simulink model "versuch2_7_3"  (R2021a)
settings: Solver=ode3  StartTime=0.0  StopTime=50  FixedStep=0.01  RelTol=1e-3
StopFcn:
  | clear con
model workspace (MAT data in the model file):
  A = Simulink.Signal
  A.DataType = 'auto'
  A.Dimensions = 1
  A.DimensionsMode = 'auto'
  A.Complexity = 'auto'
  A.SampleTime = -1
  A.SamplingMode = 'auto'
undefined symbols (not defined in the file): sigbuilder_block
libraries: simulink x11, simulink_extras x6, aerolibanimutils x1, hdlsllib x1
(part 1 of 2)
settings Model: Creator=Jan  LastModifiedBy=Oceaner
settings SolverCC: AlgebraicLoopSolver=TrustRegion
settings DataIOCC: ReturnWorkspaceOutputs=off
settings DebuggingCC: SFMachineParentedDataDiag=warning  ArithmeticOperatorsInVariantConditions=warning
settings SFSimCC: SimUseLocalCustomCode=off  CustomCodeUndefinedFunction=UseInterfaceOnly
settings RTWCC: RTWUseLocalCustomCode=off
settings CodeAppCC: StateflowObjectComments=on
settings SimscapeCC: SimscapeNormalizeSystem=off

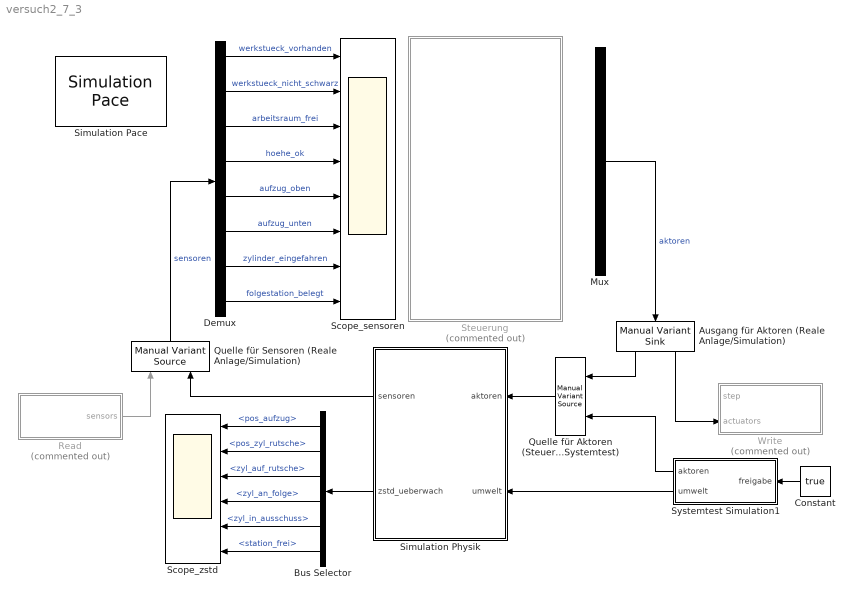
== system versuch2_7_3 ==
  " Scope_zstd" : Scope  NumInputPorts=6
  Ausgang für Aktoren (Reale Anlage/Simulation) : simulink/Signal Routing/Manual Variant Sink  NumChoices=2  LabelModeActiveChoice=V_1
  Bus Selector : BusSelector  OutputSignals=pos_aufzug,pos_zyl_rutsche,zyl_auf_rutsche,zyl_an_folge,zyl_in_ausschuss,station_frei
  Constant : Constant  Value=true
  Demux : Demux  Outputs=8
  Mux : Mux  Inputs=8
  Quelle für Aktoren (Steuerung/Systemtest) : simulink/Signal Routing/Manual Variant Source  NumChoices=2  LabelModeActiveChoice=V_2
  Quelle für Sensoren (Reale Anlage/Simulation) : simulink/Signal Routing/Manual Variant Source  NumChoices=2  LabelModeActiveChoice=V_2
  Read : Subsystem  Commented=on
  Scope_sensoren : Scope  NumInputPorts=8
  Simulation Pace : aerolibanimutils/Simulation Pace  SimulationPace=1  SleepMode=MATLAB Thread  OutputPaceError=off  SampleTime=-1
  Simulation Physik : Subsystem
  Steuerung : Stateflow chart  Commented=on  TreatAsAtomicUnit=on
  Systemtest Simulation1 : Subsystem  TreatAsAtomicUnit=on
  Write : Subsystem  Commented=on
  wires:
  Quelle für Sensoren (Reale Anlage/Simulation)/1 -> Demux/1  "sensoren"
  Read/1(sensors) -> Quelle für Sensoren (Reale Anlage/Simulation)/1
  Mux/1 -> Ausgang für Aktoren (Reale Anlage/Simulation)/1  "aktoren"
  Ausgang für Aktoren (Reale Anlage/Simulation)/2 -> Write/2(actuators)
  Ausgang für Aktoren (Reale Anlage/Simulation)/1 -> Quelle für Aktoren (Steuerung/Systemtest)/1
  Quelle für Aktoren (Steuerung/Systemtest)/1 -> Simulation Physik/1(aktoren)
  Systemtest Simulation1/1(aktoren) -> Quelle für Aktoren (Steuerung/Systemtest)/2
  Systemtest Simulation1/2(umwelt) -> Simulation Physik/2(umwelt)
  Bus Selector/1 -> " Scope_zstd"/1  "<pos_aufzug>"
  Bus Selector/2 -> " Scope_zstd"/2  "<pos_zyl_rutsche>"
  Bus Selector/3 -> " Scope_zstd"/3  "<zyl_auf_rutsche>"
  Bus Selector/4 -> " Scope_zstd"/4  "<zyl_an_folge>"
  Bus Selector/5 -> " Scope_zstd"/5  "<zyl_in_ausschuss>"
  Bus Selector/6 -> " Scope_zstd"/6  "<station_frei>"
  Demux/1 -> Scope_sensoren/1  "werkstueck_vorhanden"
  Demux/2 -> Scope_sensoren/2  "werkstueck_nicht_schwarz"
  Demux/3 -> Scope_sensoren/3  "arbeitsraum_frei"
  Demux/4 -> Scope_sensoren/4  "hoehe_ok"
  Demux/5 -> Scope_sensoren/5  "aufzug_oben"
  Demux/6 -> Scope_sensoren/6  "aufzug_unten"
  Demux/7 -> Scope_sensoren/7  "zylinder_eingefahren"
  Demux/8 -> Scope_sensoren/8  "folgestation_belegt"
  ? -> Write/1(step)  "schritt"
  Constant/1 -> Systemtest Simulation1/1(freigabe)
  Simulation Physik/1(sensoren) -> Quelle für Sensoren (Reale Anlage/Simulation)/2
  Simulation Physik/2(zstd_ueberwach) -> Bus Selector/1

== system versuch2_7_3/Read ==
  Read : MATLAB Function  TreatAsAtomicUnit=on
  sensors : Outport  VectorParamsAs1DForOutWhenUnconnected=off
  wires:
  Read/1(senarr) -> sensors/1

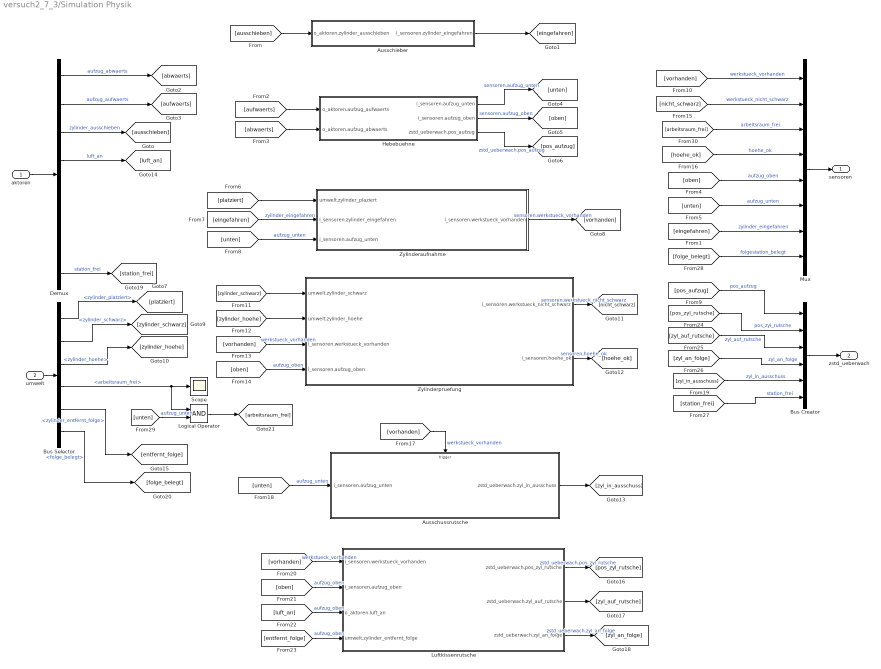
== system versuch2_7_3/Simulation Physik ==
  aktoren : Inport
  umwelt : Inport  Port=2
  Ausschieber : Subsystem
  Ausschussrutsche : Subsystem  TreatAsAtomicUnit=on
  Bus Creator : BusCreator  Inputs=6
  Bus Selector : BusSelector  OutputSignals=zylinder_platziert,zylinder_schwarz,zylinder_hoehe,arbeitsraum_frei,zylinder_entfernt_folge,folge_belegt
  Demux : Demux  Outputs=8
  Hebebuehne : Subsystem
  Logical Operator : Logic  AllPortsSameDT=off  OutDataTypeStr=boolean
  Luftkissenrutsche : Subsystem
  Mux : Mux  Inputs=8
  Scope : Scope
  Zylinderaufnahme : Subsystem
  Zylinderpruefung : Subsystem
  sensoren : Outport  VectorParamsAs1DForOutWhenUnconnected=off
  zstd_ueberwach : Outport  Port=2  VectorParamsAs1DForOutWhenUnconnected=off
  wires:
  aktoren/1 -> Demux/1
  Mux/1 -> sensoren/1
  Demux/1 -> [abwaerts]  "aufzug_abwaerts"
  [arbeitsraum_frei] -> Mux/3  "arbeitsraum_frei"
  [folge_belegt] -> Mux/8  "folgestation_belegt"
  Demux/2 -> [aufwaerts]  "aufzug_aufwaerts"
  Demux/3 -> [ausschieben]  "zylinder_ausschieben"
  [vorhanden] -> Mux/1  "werkstueck_vorhanden"
  [hoehe_ok] -> Mux/4  "hoehe_ok"
  [nicht_schwarz] -> Mux/2  "werkstueck_nicht_schwarz"
  umwelt/1 -> Bus Selector/1
  Bus Selector/1 -> [platziert]  "<zylinder_platziert>"
  Bus Selector/2 -> [zylinder_schwarz]  "<zylinder_schwarz>"
  Bus Selector/4 -> Scope/1, Logical Operator/1  "<arbeitsraum_frei>"
  Bus Selector/5 -> [entfernt_folge]  "<zylinder_entfernt_folge>"
  Bus Selector/6 -> [folge_belegt]  "<folge_belegt>"
  [pos_aufzug] -> Bus Creator/1  "pos_aufzug"
  Bus Creator/1 -> zstd_ueberwach/1
  [pos_zyl_rutsche] -> Bus Creator/2  "pos_zyl_rutsche"
  [zyl_auf_rutsche] -> Bus Creator/3  "zyl_auf_rutsche"
  [zyl_an_folge] -> Bus Creator/4  "zyl_an_folge"
  [zyl_in_ausschuss] -> Bus Creator/5  "zyl_in_ausschuss"
  [unten] -> Mux/6  "aufzug_unten"
  [eingefahren] -> Mux/7  "zylinder_eingefahren"
  [oben] -> Mux/5  "aufzug_oben"
  Bus Selector/3 -> [zylinder_hoehe]  "<zylinder_hoehe>"
  Demux/8 -> [station_frei]  "station_frei"
  [station_frei] -> Bus Creator/6  "station_frei"
  [ausschieben] -> Ausschieber/1(o_aktoren.zylinder_ausschieben)
  Ausschieber/1(i_sensoren.zylinder_eingefahren) -> [eingefahren]
  [aufwaerts] -> Hebebuehne/1(o_aktoren.aufzug_aufwaerts)
  [abwaerts] -> Hebebuehne/2(o_aktoren.aufzug_abwaerts)
  Hebebuehne/1(i_sensoren.aufzug_unten) -> [unten]  "sensoren.aufzug_unten"
  Hebebuehne/2(i_sensoren.aufzug_oben) -> [oben]  "sensoren.aufzug_oben"
  Hebebuehne/3(zstd_ueberwach.pos_aufzug) -> [pos_aufzug]  "zstd_ueberwach.pos_aufzug"
  [platziert] -> Zylinderaufnahme/1(umwelt.zylinder_plaziert)
  [eingefahren] -> Zylinderaufnahme/2(i_sensoren.zylinder_eingefahren)  "zylinder_eingefahren"
  [unten] -> Zylinderaufnahme/3(i_sensoren.aufzug_unten)  "aufzug_unten"
  Zylinderaufnahme/1(i_sensoren.werkstueck_vorhanden) -> [vorhanden]  "sensoren.werkstueck_vorhanden"
  [vorhanden] -> Ausschussrutsche/Trigger  "werkstueck_vorhanden"
  [unten] -> Ausschussrutsche/1(i_sensoren.aufzug_unten)  "aufzug_unten"
  Ausschussrutsche/1(zstd_ueberwach.zyl_in_ausschuss) -> [zyl_in_ausschuss]
  [vorhanden] -> Luftkissenrutsche/1(i_sensoren.werkstueck_vorhanden)  "werkstueck_vorhanden"
  [oben] -> Luftkissenrutsche/2(i_sensoren.aufzug_oben)  "aufzug_oben"
  Demux/4 -> [luft_an]  "luft_an"
  [luft_an] -> Luftkissenrutsche/3(o_aktoren.luft_an)  "aufzug_oben"
  [entfernt_folge] -> Luftkissenrutsche/4(umwelt.zylinder_entfernt_folge)  "aufzug_oben"
  Luftkissenrutsche/1(zstd_ueberwach.pos_zyl_rutsche) -> [pos_zyl_rutsche]  "zstd_ueberwach.pos_zyl_rutsche"
  Luftkissenrutsche/2(zstd_ueberwach.zyl_auf_rutsche) -> [zyl_auf_rutsche]
  Luftkissenrutsche/3(zstd_ueberwach.zyl_an_folge) -> [zyl_an_folge]  "zstd_ueberwach.zyl_an_folge"
  [unten] -> Logical Operator/2  "aufzug_unten"
  Logical Operator/1 -> [arbeitsraum_frei]
  Zylinderpruefung/1(i_sensoren.werkstueck_nicht_schwarz) -> [nicht_schwarz]  "sensoren.werkstueck_nicht_schwarz"
  [zylinder_hoehe] -> Zylinderpruefung/2(umwelt.zylinder_hoehe)
  [oben] -> Zylinderpruefung/4(i_sensoren.aufzug_oben)  "aufzug_oben"
  [vorhanden] -> Zylinderpruefung/3(i_sensoren.werkstueck_vorhanden)  "werkstueck_vorhanden"
  [zylinder_schwarz] -> Zylinderpruefung/1(umwelt.zylinder_schwarz)
  Zylinderpruefung/2(i_sensoren.hoehe_ok) -> [hoehe_ok]  "sensoren.hoehe_ok"

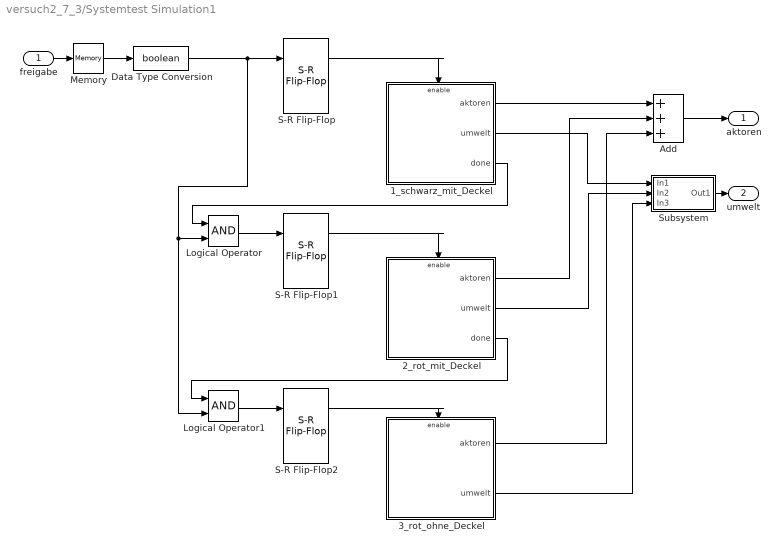
== system versuch2_7_3/Systemtest Simulation1 ==
  freigabe : Inport
  1_schwarz_mit_Deckel : Subsystem
  2_rot_mit_Deckel : Subsystem
  3_rot_ohne_Deckel : Subsystem
  Add : Sum  Inputs=+++
  Data Type Conversion : DataTypeConversion  OutDataTypeStr=boolean
  Logical Operator : Logic  AllPortsSameDT=off  OutDataTypeStr=boolean
  Logical Operator1 : Logic  AllPortsSameDT=off  OutDataTypeStr=boolean
  Memory : Memory
  S-R Flip-Flop : simulink_extras/Flip Flops/S-R Flip-Flop  initial_condition=0
  S-R Flip-Flop1 : simulink_extras/Flip Flops/S-R Flip-Flop  initial_condition=0
  S-R Flip-Flop2 : simulink_extras/Flip Flops/S-R Flip-Flop  initial_condition=0
  Subsystem : Subsystem
  aktoren : Outport  VectorParamsAs1DForOutWhenUnconnected=off
  umwelt : Outport  Port=2  VectorParamsAs1DForOutWhenUnconnected=off
  wires:
  freigabe/1 -> Memory/1
  S-R Flip-Flop/1 -> 1_schwarz_mit_Deckel/Enable
  Logical Operator/1 -> S-R Flip-Flop1/1
  1_schwarz_mit_Deckel/3(done) -> Logical Operator/1
  S-R Flip-Flop1/1 -> 2_rot_mit_Deckel/Enable
  Logical Operator1/1 -> S-R Flip-Flop2/1
  2_rot_mit_Deckel/3(done) -> Logical Operator1/1
  S-R Flip-Flop2/1 -> 3_rot_ohne_Deckel/Enable
  1_schwarz_mit_Deckel/1(aktoren) -> Add/1
  2_rot_mit_Deckel/1(aktoren) -> Add/2
  Add/1 -> aktoren/1
  3_rot_ohne_Deckel/1(aktoren) -> Add/3
  Subsystem/1(Out1) -> umwelt/1
  1_schwarz_mit_Deckel/2(umwelt) -> Subsystem/1(In1)
  2_rot_mit_Deckel/2(umwelt) -> Subsystem/2(In2)
  3_rot_ohne_Deckel/2(umwelt) -> Subsystem/3(In3)
  Data Type Conversion/1 -> Logical Operator1/2, Logical Operator/2, S-R Flip-Flop/1
  Memory/1 -> Data Type Conversion/1

== system versuch2_7_3/Write ==
  step : Inport
  actuators : Inport  Port=2
  Data Type Conversion : DataTypeConversion  OutDataTypeStr=boolean
  Write1 : MATLAB Function  TreatAsAtomicUnit=on
  wires:
  step/1 -> Write1/1(step)
  Data Type Conversion/1 -> Write1/2(actuators)
  actuators/1 -> Data Type Conversion/1

== system versuch2_7_3/Simulation Physik/Ausschieber ==
  o_aktoren.zylinder_ausschieben : Inport
  Delay : Delay  DelayLength=50  InitialCondition=0
  Logical Operator : Logic  Operator=NOT  AllPortsSameDT=off  OutDataTypeStr=boolean
  Scope : Scope  NumInputPorts=2
  i_sensoren.zylinder_eingefahren : Outport
  wires:
  o_aktoren.zylinder_ausschieben/1 -> Logical Operator/1, Scope/2  "aktoren.zylinder_ausschieben"
  Delay/1 -> Scope/1, i_sensoren.zylinder_eingefahren/1  "sensoren.zylinder_eingefahren"
  Logical Operator/1 -> Delay/1

== system versuch2_7_3/Simulation Physik/Ausschussrutsche ==
  i_sensoren.aufzug_unten : Inport
  i_sensoren.werkstueck_vorhanden : TriggerPort  TriggerType=falling  VariantControl=(inherit)
  Add : Sum
  Constant : Constant
  Data Type Conversion : DataTypeConversion  OutDataTypeStr=double
  Logical Operator : Logic  AllPortsSameDT=off  OutDataTypeStr=boolean
  Memory1 : Memory  InheritSampleTime=on
  zstd_ueberwach.zyl_in_ausschuss : Outport
  wires:
  Add/1 -> zstd_ueberwach.zyl_in_ausschuss/1, Memory1/1
  Constant/1 -> Logical Operator/2
  Memory1/1 -> Add/2
  i_sensoren.aufzug_unten/1 -> Logical Operator/1
  Logical Operator/1 -> Data Type Conversion/1
  Data Type Conversion/1 -> Add/1

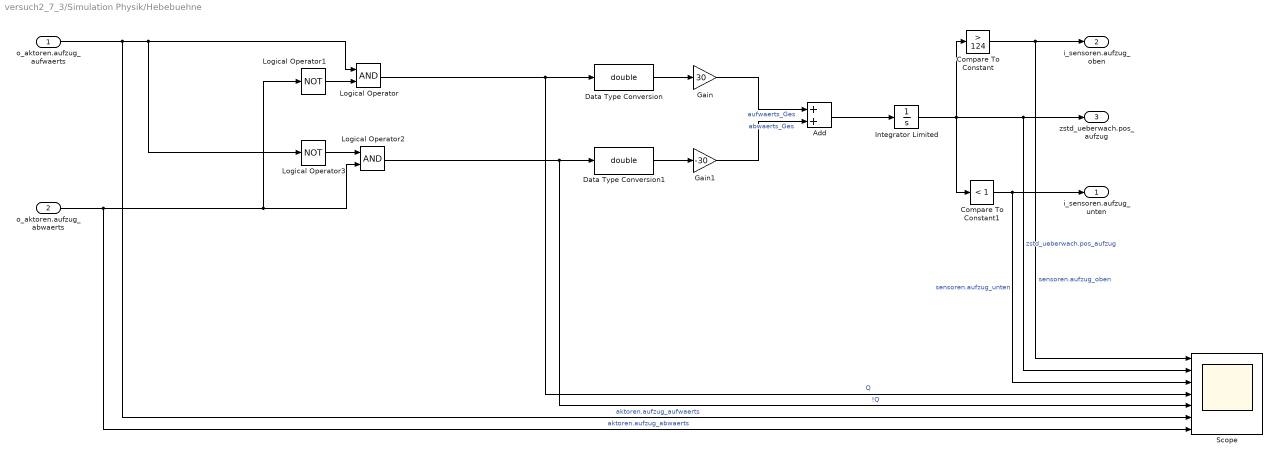
== system versuch2_7_3/Simulation Physik/Hebebuehne ==
  o_aktoren.aufzug_aufwaerts : Inport
  o_aktoren.aufzug_abwaerts : Inport  Port=2
  Add : Sum
  Compare To Constant : simulink/Logic and Bit Operations/Compare To Constant  relop=>  const=124  OutDataTypeStr=boolean
  Compare To Constant1 : simulink/Logic and Bit Operations/Compare To Constant  relop=<  const=1  OutDataTypeStr=boolean
  Data Type Conversion : DataTypeConversion  OutDataTypeStr=double
  Data Type Conversion1 : DataTypeConversion  OutDataTypeStr=double
  Gain : Gain  Gain=30
  Gain1 : Gain  Gain=-30
  Integrator Limited : Integrator  LimitOutput=on  UpperSaturationLimit=125  LowerSaturationLimit=0
  Logical Operator : Logic  AllPortsSameDT=off  OutDataTypeStr=boolean
  Logical Operator1 : Logic  Operator=NOT  AllPortsSameDT=off  OutDataTypeStr=boolean
  Logical Operator2 : Logic  AllPortsSameDT=off  OutDataTypeStr=boolean
  Logical Operator3 : Logic  Operator=NOT  AllPortsSameDT=off  OutDataTypeStr=boolean
  Scope : Scope  NumInputPorts=7
  i_sensoren.aufzug_unten : Outport
  i_sensoren.aufzug_oben : Outport  Port=2
  zstd_ueberwach.pos_aufzug : Outport  Port=3
  wires:
  Logical Operator/1 -> Data Type Conversion/1, Scope/4  "Q"
  Gain/1 -> Add/1  "aufwaerts_Ges"
  Logical Operator2/1 -> Data Type Conversion1/1, Scope/5  "!Q"
  Gain1/1 -> Add/2  "abwaerts_Ges"
  Integrator Limited/1 -> Compare To Constant/1, Compare To Constant1/1, Scope/2, zstd_ueberwach.pos_aufzug/1  "zstd_ueberwach.pos_aufzug"
  Compare To Constant/1 -> Scope/1, i_sensoren.aufzug_oben/1  "sensoren.aufzug_oben"
  Compare To Constant1/1 -> Scope/3, i_sensoren.aufzug_unten/1  "sensoren.aufzug_unten"
  o_aktoren.aufzug_aufwaerts/1 -> Scope/6, Logical Operator3/1, Logical Operator/1  "aktoren.aufzug_aufwaerts"
  o_aktoren.aufzug_abwaerts/1 -> Scope/7, Logical Operator2/2, Logical Operator1/1  "aktoren.aufzug_abwaerts"
  Logical Operator1/1 -> Logical Operator/2
  Logical Operator3/1 -> Logical Operator2/1
  Data Type Conversion/1 -> Gain/1
  Data Type Conversion1/1 -> Gain1/1
  Add/1 -> Integrator Limited/1

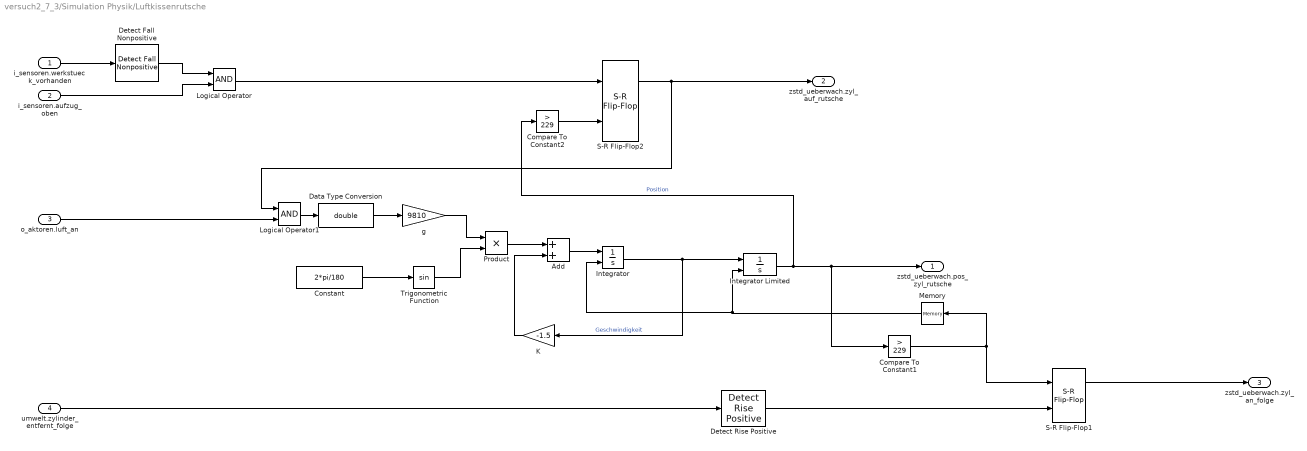
== system versuch2_7_3/Simulation Physik/Luftkissenrutsche ==
  i_sensoren.werkstueck_vorhanden : Inport
  i_sensoren.aufzug_oben : Inport  Port=2
  o_aktoren.luft_an : Inport  Port=3
  umwelt.zylinder_entfernt_folge : Inport  Port=4
  Add : Sum
  Compare To Constant1 : simulink/Logic and Bit Operations/Compare To Constant  relop=>  const=229  OutDataTypeStr=boolean
  Compare To Constant2 : simulink/Logic and Bit Operations/Compare To Constant  relop=>  const=229  OutDataTypeStr=boolean
  Constant : Constant  Value=2*pi/180
  Data Type Conversion : DataTypeConversion  OutDataTypeStr=double
  Detect Fall Nonpositive : simulink/Logic and Bit Operations/Detect Fall Nonpositive  vinit=0  OutDataTypeStr=boolean
      settings: SourceProductBaseCode=SL
  Detect Rise Positive : simulink/Logic and Bit Operations/Detect Rise Positive  vinit=0  OutDataTypeStr=boolean
  Integrator : Integrator  ExternalReset=rising
  Integrator Limited : Integrator  ExternalReset=rising  LimitOutput=on  UpperSaturationLimit=230  LowerSaturationLimit=0
  K : Gain  Gain=-1.5
  Logical Operator : Logic  AllPortsSameDT=off  OutDataTypeStr=boolean
  Logical Operator1 : Logic  AllPortsSameDT=off  OutDataTypeStr=boolean
  Memory : Memory
  Product : Product
  S-R Flip-Flop1 : simulink_extras/Flip Flops/S-R Flip-Flop  initial_condition=0
  S-R Flip-Flop2 : simulink_extras/Flip Flops/S-R Flip-Flop  initial_condition=0
  Trigonometric Function : Trigonometry
  g : Gain  Gain=9810
  zstd_ueberwach.pos_zyl_rutsche : Outport
  zstd_ueberwach.zyl_auf_rutsche : Outport  Port=2
  zstd_ueberwach.zyl_an_folge : Outport  Port=3
  wires:
  i_sensoren.aufzug_oben/1 -> Logical Operator/2
  i_sensoren.werkstueck_vorhanden/1 -> Detect Fall Nonpositive/1
  Detect Fall Nonpositive/1 -> Logical Operator/1
  Logical Operator/1 -> S-R Flip-Flop2/1
  o_aktoren.luft_an/1 -> Logical Operator1/2
  Logical Operator1/1 -> Data Type Conversion/1
  Data Type Conversion/1 -> g/1
  Constant/1 -> Trigonometric Function/1
  g/1 -> Product/1
  Trigonometric Function/1 -> Product/2
  Product/1 -> Add/1
  Add/1 -> Integrator/1
  Integrator/1 -> Integrator Limited/1, K/1  "Geschwindigkeit"
  K/1 -> Add/2
  Integrator Limited/1 -> Compare To Constant1/1, zstd_ueberwach.pos_zyl_rutsche/1, Compare To Constant2/1  "Position"
  Compare To Constant1/1 -> S-R Flip-Flop1/1, Memory/1
  S-R Flip-Flop2/1 -> Logical Operator1/1, zstd_ueberwach.zyl_auf_rutsche/1
  Memory/1 -> Integrator/2, Integrator Limited/2
  S-R Flip-Flop1/1 -> zstd_ueberwach.zyl_an_folge/1
  umwelt.zylinder_entfernt_folge/1 -> Detect Rise Positive/1
  Detect Rise Positive/1 -> S-R Flip-Flop1/2
  Compare To Constant2/1 -> S-R Flip-Flop2/2

== system versuch2_7_3/Simulation Physik/Zylinderaufnahme ==
  umwelt.zylinder_plaziert : Inport
  i_sensoren.zylinder_eingefahren : Inport  Port=2
  i_sensoren.aufzug_unten : Inport  Port=3
  Detect Fall Nonpositive : simulink/Logic and Bit Operations/Detect Fall Nonpositive  vinit=0  OutDataTypeStr=boolean
      settings: SourceProductBaseCode=SL
  Detect Rise Positive : simulink/Logic and Bit Operations/Detect Rise Positive  vinit=0  OutDataTypeStr=boolean
  Logical Operator1 : Logic  Inputs=3  AllPortsSameDT=off  OutDataTypeStr=boolean
  S-R Flip-Flop : simulink_extras/Flip Flops/S-R Flip-Flop  initial_condition=0
  Scope : Scope  NumInputPorts=4
  i_sensoren.werkstueck_vorhanden : Outport
  wires:
  i_sensoren.zylinder_eingefahren/1 -> Scope/3, Logical Operator1/3, Detect Fall Nonpositive/1
  i_sensoren.aufzug_unten/1 -> Logical Operator1/2, Scope/2
  umwelt.zylinder_plaziert/1 -> Scope/1, Detect Rise Positive/1
  Logical Operator1/1 -> S-R Flip-Flop/1
  S-R Flip-Flop/1 -> Scope/4, i_sensoren.werkstueck_vorhanden/1
  Detect Fall Nonpositive/1 -> S-R Flip-Flop/2
  Detect Rise Positive/1 -> Logical Operator1/1

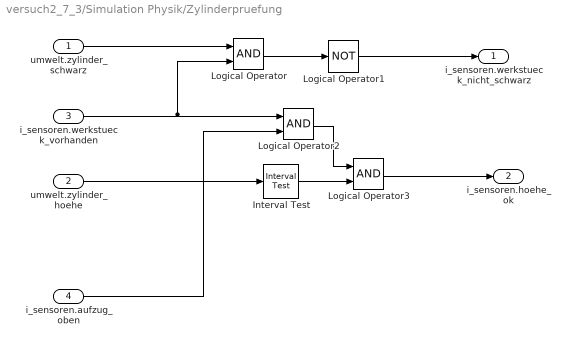
== system versuch2_7_3/Simulation Physik/Zylinderpruefung ==
  umwelt.zylinder_schwarz : Inport
  umwelt.zylinder_hoehe : Inport  Port=2
  i_sensoren.werkstueck_vorhanden : Inport  Port=3
  i_sensoren.aufzug_oben : Inport  Port=4
  Interval Test : hdlsllib/Logic and Bit Operations/Interval Test  IntervalClosedRight=on  uplimit=26  IntervalClosedLeft=on  lowlimit=24  OutDataTypeStr=boolean
      settings: SourceProductBaseCode=SL
  Logical Operator : Logic  AllPortsSameDT=off  OutDataTypeStr=boolean
  Logical Operator1 : Logic  Operator=NOT  AllPortsSameDT=off  OutDataTypeStr=boolean
  Logical Operator2 : Logic  AllPortsSameDT=off  OutDataTypeStr=boolean
  Logical Operator3 : Logic  AllPortsSameDT=off  OutDataTypeStr=boolean
  i_sensoren.werkstueck_nicht_schwarz : Outport
  i_sensoren.hoehe_ok : Outport  Port=2
  wires:
  umwelt.zylinder_schwarz/1 -> Logical Operator/1
  Logical Operator/1 -> Logical Operator1/1
  i_sensoren.werkstueck_vorhanden/1 -> Logical Operator2/1, Logical Operator/2
  Logical Operator1/1 -> i_sensoren.werkstueck_nicht_schwarz/1
  i_sensoren.aufzug_oben/1 -> Logical Operator2/2
  umwelt.zylinder_hoehe/1 -> Interval Test/1
  Interval Test/1 -> Logical Operator3/2
  Logical Operator2/1 -> Logical Operator3/1
  Logical Operator3/1 -> i_sensoren.hoehe_ok/1

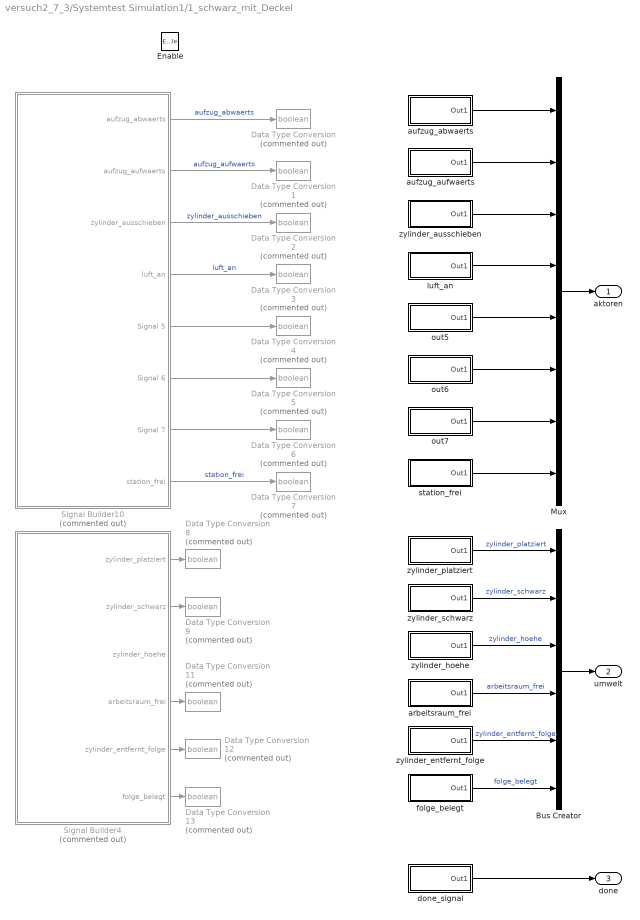
== system versuch2_7_3/Systemtest Simulation1/1_schwarz_mit_Deckel ==
  Enable : EnablePort
  Bus Creator : BusCreator  Inputs=6
  Data Type Conversion{,1..9,11..13} (13 alike) : DataTypeConversion  Commented=on  OutDataTypeStr=boolean
  Mux : Mux  Inputs=8
  Signal Builder10 : Subsystem  Tag=STV Subsys  Commented=on  LoadFcn=sigbuilder_block('load');  StartFcn=sigbuilder_block('start');  StopFcn=sigbuilder_block('stop');  ClipboardFcn=sigbuilder_block('clipboard');  mask(Sigbuilder block){tuvar=[0:10]}
      mask help: Simulink:masks:SigbuilderBlock_MD
      mask init:
      | if ~strcmp(get_param(bdroot(gcbh),'SimulationStatus'),'stopped') tuvar = sigbuilder_block('maskInit'); end
      settings: CopyFcn=sigbuilder_block('copy');  DeleteFcn=sigbuilder_block('delete');  ModelCloseFcn=sigbuilder_block('modelClose');  PreSaveFcn=sigbuilder_block('preSave');  PauseFcn=sigbuilder_block('pause');  ContinueFcn=sigbuilder_block('continue');  NameChangeFcn=sigbuilder_block('namechange');  OpenFcn=sigbuilder_block('open',[2160 -195 1440 817.5 ]);  CloseFcn=sigbuilder_block('close');
      mask Display: plot(0, 0, 100, 100,[2, 2, 32, 32, 2], [68, 8, 8, 68, 68],[32, 2], [38, 38], [32, 19, 2],[53, 60, 44], [32, 17, 17, 2],[16, 16, 31, 31]);txt = getActiveGroup(gcbh);text(2, 100, txt,'verticalAlignment', 'top');
  Signal Builder4 : Subsystem  Tag=STV Subsys  Commented=on  LoadFcn=sigbuilder_block('load');  StartFcn=sigbuilder_block('start');  StopFcn=sigbuilder_block('stop');  ClipboardFcn=sigbuilder_block('clipboard');  mask(Sigbuilder block){tuvar=[0:10]}
      mask help: Simulink:masks:SigbuilderBlock_MD
      mask init:
      | if ~strcmp(get_param(bdroot(gcbh),'SimulationStatus'),'stopped') tuvar = sigbuilder_block('maskInit'); end
      settings: CopyFcn=sigbuilder_block('copy');  DeleteFcn=sigbuilder_block('delete');  ModelCloseFcn=sigbuilder_block('modelClose');  PreSaveFcn=sigbuilder_block('preSave');  PauseFcn=sigbuilder_block('pause');  ContinueFcn=sigbuilder_block('continue');  NameChangeFcn=sigbuilder_block('namechange');  OpenFcn=sigbuilder_block('open',[4.875 4.875 1070.25 612.75 ]);  CloseFcn=sigbuilder_block('close');
      mask Display: plot(0, 0, 100, 100,[2, 2, 32, 32, 2], [68, 8, 8, 68, 68],[32, 2], [38, 38], [32, 19, 2],[53, 60, 44], [32, 17, 17, 2],[16, 16, 31, 31]);txt = getActiveGroup(gcbh);text(2, 100, txt,'verticalAlignment', 'top');
  arbeitsraum_frei : Subsystem
  aufzug_abwaerts : Subsystem
  aufzug_aufwaerts : Subsystem
  done_signal : Subsystem
  folge_belegt : Subsystem
  luft_an : Subsystem
  out5 : Subsystem
  out6 : Subsystem
  out7 : Subsystem
  station_frei : Subsystem
  zylinder_ausschieben : Subsystem
  zylinder_entfernt_folge : Subsystem
  zylinder_hoehe : Subsystem
  zylinder_platziert : Subsystem
  zylinder_schwarz : Subsystem
  aktoren : Outport  VectorParamsAs1DForOutWhenUnconnected=off
  umwelt : Outport  Port=2  VectorParamsAs1DForOutWhenUnconnected=off
  done : Outport  Port=3  VectorParamsAs1DForOutWhenUnconnected=off
  wires:
  Bus Creator/1 -> umwelt/1
  Signal Builder4/1(zylinder_platziert) -> Data Type Conversion8/1
  Signal Builder4/2(zylinder_schwarz) -> Data Type Conversion9/1
  zylinder_hoehe/1(Out1) -> Bus Creator/3  "zylinder_hoehe"
  Signal Builder4/4(arbeitsraum_frei) -> Data Type Conversion11/1
  Signal Builder4/5(zylinder_entfernt_folge) -> Data Type Conversion12/1
  Signal Builder4/6(folge_belegt) -> Data Type Conversion13/1
  zylinder_platziert/1(Out1) -> Bus Creator/1  "zylinder_platziert"
  zylinder_schwarz/1(Out1) -> Bus Creator/2  "zylinder_schwarz"
  arbeitsraum_frei/1(Out1) -> Bus Creator/4  "arbeitsraum_frei"
  zylinder_entfernt_folge/1(Out1) -> Bus Creator/5  "zylinder_entfernt_folge"
  folge_belegt/1(Out1) -> Bus Creator/6  "folge_belegt"
  Mux/1 -> aktoren/1
  Signal Builder10/1(aufzug_abwaerts) -> Data Type Conversion/1  "aufzug_abwaerts"
  Signal Builder10/2(aufzug_aufwaerts) -> Data Type Conversion1/1  "aufzug_aufwaerts"
  Signal Builder10/3(zylinder_ausschieben) -> Data Type Conversion2/1  "zylinder_ausschieben"
  Signal Builder10/4(luft_an) -> Data Type Conversion3/1  "luft_an"
  Signal Builder10/8(station_frei) -> Data Type Conversion7/1  "station_frei"
  Signal Builder10/5(Signal 5) -> Data Type Conversion4/1
  Signal Builder10/6(Signal 6) -> Data Type Conversion5/1
  Signal Builder10/7(Signal 7) -> Data Type Conversion6/1
  aufzug_abwaerts/1(Out1) -> Mux/1
  aufzug_aufwaerts/1(Out1) -> Mux/2
  zylinder_ausschieben/1(Out1) -> Mux/3
  luft_an/1(Out1) -> Mux/4
  out5/1(Out1) -> Mux/5
  out6/1(Out1) -> Mux/6
  out7/1(Out1) -> Mux/7
  station_frei/1(Out1) -> Mux/8
  done_signal/1(Out1) -> done/1

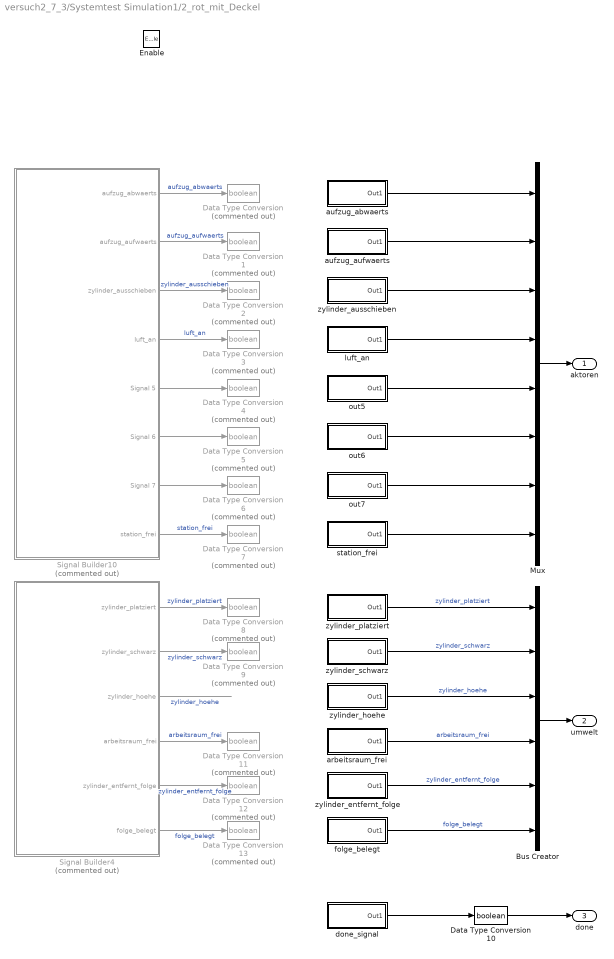
== system versuch2_7_3/Systemtest Simulation1/2_rot_mit_Deckel ==
  Enable : EnablePort
  Bus Creator : BusCreator  Inputs=6
  Data Type Conversion{,1..9,11..13} (13 alike) : DataTypeConversion  Commented=on  OutDataTypeStr=boolean
  Data Type Conversion10 : DataTypeConversion  OutDataTypeStr=boolean
  Mux : Mux  Inputs=8
  Signal Builder10 : Subsystem  Tag=STV Subsys  Commented=on  LoadFcn=sigbuilder_block('load');  StartFcn=sigbuilder_block('start');  StopFcn=sigbuilder_block('stop');  ClipboardFcn=sigbuilder_block('clipboard');  mask(Sigbuilder block){tuvar=[0:10]}
      mask help: Simulink:masks:SigbuilderBlock_MD
      mask init:
      | if ~strcmp(get_param(bdroot(gcbh),'SimulationStatus'),'stopped') tuvar = sigbuilder_block('maskInit'); end
      settings: CopyFcn=sigbuilder_block('copy');  DeleteFcn=sigbuilder_block('delete');  ModelCloseFcn=sigbuilder_block('modelClose');  PreSaveFcn=sigbuilder_block('preSave');  PauseFcn=sigbuilder_block('pause');  ContinueFcn=sigbuilder_block('continue');  NameChangeFcn=sigbuilder_block('namechange');  OpenFcn=sigbuilder_block('open',[4.875 4.875 1070.25 612.75 ]);  CloseFcn=sigbuilder_block('close');
      mask Display: plot(0, 0, 100, 100,[2, 2, 32, 32, 2], [68, 8, 8, 68, 68],[32, 2], [38, 38], [32, 19, 2],[53, 60, 44], [32, 17, 17, 2],[16, 16, 31, 31]);txt = getActiveGroup(gcbh);text(2, 100, txt,'verticalAlignment', 'top');
  Signal Builder4 : Subsystem  Tag=STV Subsys  Commented=on  LoadFcn=sigbuilder_block('load');  StartFcn=sigbuilder_block('start');  StopFcn=sigbuilder_block('stop');  ClipboardFcn=sigbuilder_block('clipboard');  mask(Sigbuilder block){tuvar=[0:10]}
      mask help: Simulink:masks:SigbuilderBlock_MD
      mask init:
      | if ~strcmp(get_param(bdroot(gcbh),'SimulationStatus'),'stopped') tuvar = sigbuilder_block('maskInit'); end
      settings: CopyFcn=sigbuilder_block('copy');  DeleteFcn=sigbuilder_block('delete');  ModelCloseFcn=sigbuilder_block('modelClose');  PreSaveFcn=sigbuilder_block('preSave');  PauseFcn=sigbuilder_block('pause');  ContinueFcn=sigbuilder_block('continue');  NameChangeFcn=sigbuilder_block('namechange');  OpenFcn=sigbuilder_block('open',[2160 -195 1440 817.5 ]);  CloseFcn=sigbuilder_block('close');
      mask Display: plot(0, 0, 100, 100,[2, 2, 32, 32, 2], [68, 8, 8, 68, 68],[32, 2], [38, 38], [32, 19, 2],[53, 60, 44], [32, 17, 17, 2],[16, 16, 31, 31]);txt = getActiveGroup(gcbh);text(2, 100, txt,'verticalAlignment', 'top');
  arbeitsraum_frei : Subsystem
  aufzug_abwaerts : Subsystem
  aufzug_aufwaerts : Subsystem
  done_signal : Subsystem
  folge_belegt : Subsystem
  luft_an : Subsystem
  out5 : Subsystem
  out6 : Subsystem
  out7 : Subsystem
  station_frei : Subsystem
  zylinder_ausschieben : Subsystem
  zylinder_entfernt_folge : Subsystem
  zylinder_hoehe : Subsystem
  zylinder_platziert : Subsystem
  zylinder_schwarz : Subsystem
  aktoren : Outport  VectorParamsAs1DForOutWhenUnconnected=off
  umwelt : Outport  Port=2  VectorParamsAs1DForOutWhenUnconnected=off
  done : Outport  Port=3  VectorParamsAs1DForOutWhenUnconnected=off
  wires:
  Bus Creator/1 -> umwelt/1
  Signal Builder4/1(zylinder_platziert) -> Data Type Conversion8/1  "zylinder_platziert"
  Signal Builder4/2(zylinder_schwarz) -> Data Type Conversion9/1  "zylinder_schwarz"
  Signal Builder4/3(zylinder_hoehe) -> ?  "zylinder_hoehe"
  Signal Builder4/4(arbeitsraum_frei) -> Data Type Conversion11/1  "arbeitsraum_frei"
  Signal Builder4/5(zylinder_entfernt_folge) -> Data Type Conversion12/1  "zylinder_entfernt_folge"
  Signal Builder4/6(folge_belegt) -> Data Type Conversion13/1  "folge_belegt"
  zylinder_platziert/1(Out1) -> Bus Creator/1  "zylinder_platziert"
  zylinder_schwarz/1(Out1) -> Bus Creator/2  "zylinder_schwarz"
  arbeitsraum_frei/1(Out1) -> Bus Creator/4  "arbeitsraum_frei"
  zylinder_entfernt_folge/1(Out1) -> Bus Creator/5  "zylinder_entfernt_folge"
  folge_belegt/1(Out1) -> Bus Creator/6  "folge_belegt"
  Mux/1 -> aktoren/1
  Signal Builder10/1(aufzug_abwaerts) -> Data Type Conversion/1  "aufzug_abwaerts"
  Signal Builder10/2(aufzug_aufwaerts) -> Data Type Conversion1/1  "aufzug_aufwaerts"
  Signal Builder10/3(zylinder_ausschieben) -> Data Type Conversion2/1  "zylinder_ausschieben"
  Signal Builder10/4(luft_an) -> Data Type Conversion3/1  "luft_an"
  Signal Builder10/8(station_frei) -> Data Type Conversion7/1  "station_frei"
  Signal Builder10/5(Signal 5) -> Data Type Conversion4/1
  Signal Builder10/6(Signal 6) -> Data Type Conversion5/1
  Signal Builder10/7(Signal 7) -> Data Type Conversion6/1
  aufzug_abwaerts/1(Out1) -> Mux/1
  aufzug_aufwaerts/1(Out1) -> Mux/2
  zylinder_ausschieben/1(Out1) -> Mux/3
  luft_an/1(Out1) -> Mux/4
  out5/1(Out1) -> Mux/5
  out6/1(Out1) -> Mux/6
  out7/1(Out1) -> Mux/7
  station_frei/1(Out1) -> Mux/8
  Data Type Conversion10/1 -> done/1
  done_signal/1(Out1) -> Data Type Conversion10/1
  zylinder_hoehe/1(Out1) -> Bus Creator/3  "zylinder_hoehe"

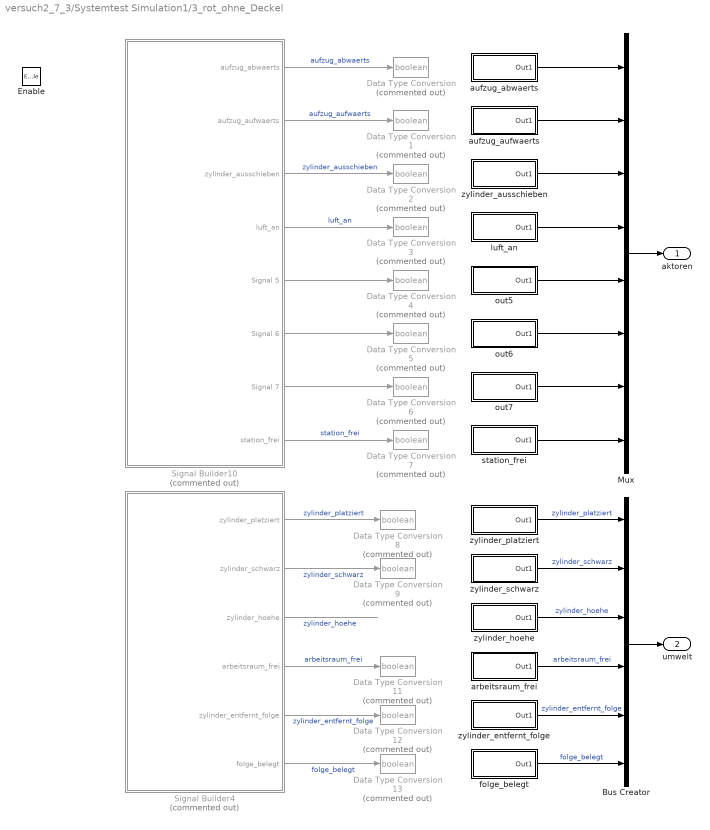
== system versuch2_7_3/Systemtest Simulation1/3_rot_ohne_Deckel ==
  Enable : EnablePort
  Bus Creator : BusCreator  Inputs=6
  Data Type Conversion{,1..9,11..13} (13 alike) : DataTypeConversion  Commented=on  OutDataTypeStr=boolean
  Mux : Mux  Inputs=8
  Signal Builder10 : Subsystem  Tag=STV Subsys  Commented=on  LoadFcn=sigbuilder_block('load');  StartFcn=sigbuilder_block('start');  StopFcn=sigbuilder_block('stop');  ClipboardFcn=sigbuilder_block('clipboard');  mask(Sigbuilder block){tuvar=[0:10]}
      mask help: Simulink:masks:SigbuilderBlock_MD
      mask init:
      | if ~strcmp(get_param(bdroot(gcbh),'SimulationStatus'),'stopped') tuvar = sigbuilder_block('maskInit'); end
      settings: CopyFcn=sigbuilder_block('copy');  DeleteFcn=sigbuilder_block('delete');  ModelCloseFcn=sigbuilder_block('modelClose');  PreSaveFcn=sigbuilder_block('preSave');  PauseFcn=sigbuilder_block('pause');  ContinueFcn=sigbuilder_block('continue');  NameChangeFcn=sigbuilder_block('namechange');  OpenFcn=sigbuilder_block('open',[2160 -195 1440 817.5 ]);  CloseFcn=sigbuilder_block('close');
      mask Display: plot(0, 0, 100, 100,[2, 2, 32, 32, 2], [68, 8, 8, 68, 68],[32, 2], [38, 38], [32, 19, 2],[53, 60, 44], [32, 17, 17, 2],[16, 16, 31, 31]);txt = getActiveGroup(gcbh);text(2, 100, txt,'verticalAlignment', 'top');
  Signal Builder4 : Subsystem  Tag=STV Subsys  Commented=on  LoadFcn=sigbuilder_block('load');  StartFcn=sigbuilder_block('start');  StopFcn=sigbuilder_block('stop');  ClipboardFcn=sigbuilder_block('clipboard');  mask(Sigbuilder block){tuvar=[0:10]}
      mask help: Simulink:masks:SigbuilderBlock_MD
      mask init:
      | if ~strcmp(get_param(bdroot(gcbh),'SimulationStatus'),'stopped') tuvar = sigbuilder_block('maskInit'); end
      settings: CopyFcn=sigbuilder_block('copy');  DeleteFcn=sigbuilder_block('delete');  ModelCloseFcn=sigbuilder_block('modelClose');  PreSaveFcn=sigbuilder_block('preSave');  PauseFcn=sigbuilder_block('pause');  ContinueFcn=sigbuilder_block('continue');  NameChangeFcn=sigbuilder_block('namechange');  OpenFcn=sigbuilder_block('open',[2160 -195 1440 817.5 ]);  CloseFcn=sigbuilder_block('close');
      mask Display: plot(0, 0, 100, 100,[2, 2, 32, 32, 2], [68, 8, 8, 68, 68],[32, 2], [38, 38], [32, 19, 2],[53, 60, 44], [32, 17, 17, 2],[16, 16, 31, 31]);txt = getActiveGroup(gcbh);text(2, 100, txt,'verticalAlignment', 'top');
  arbeitsraum_frei : Subsystem
  aufzug_abwaerts : Subsystem
  aufzug_aufwaerts : Subsystem
  folge_belegt : Subsystem
  luft_an : Subsystem
  out5 : Subsystem
  out6 : Subsystem
  out7 : Subsystem
  station_frei : Subsystem
  zylinder_ausschieben : Subsystem
  zylinder_entfernt_folge : Subsystem
  zylinder_hoehe : Subsystem
  zylinder_platziert : Subsystem
  zylinder_schwarz : Subsystem
  aktoren : Outport  VectorParamsAs1DForOutWhenUnconnected=off
  umwelt : Outport  Port=2  VectorParamsAs1DForOutWhenUnconnected=off
  wires:
  Bus Creator/1 -> umwelt/1
  Signal Builder4/1(zylinder_platziert) -> Data Type Conversion8/1  "zylinder_platziert"
  Signal Builder4/2(zylinder_schwarz) -> Data Type Conversion9/1  "zylinder_schwarz"
  Signal Builder4/3(zylinder_hoehe) -> ?  "zylinder_hoehe"
  Signal Builder4/4(arbeitsraum_frei) -> Data Type Conversion11/1  "arbeitsraum_frei"
  Signal Builder4/5(zylinder_entfernt_folge) -> Data Type Conversion12/1  "zylinder_entfernt_folge"
  Signal Builder4/6(folge_belegt) -> Data Type Conversion13/1  "folge_belegt"
  zylinder_platziert/1(Out1) -> Bus Creator/1  "zylinder_platziert"
  zylinder_schwarz/1(Out1) -> Bus Creator/2  "zylinder_schwarz"
  arbeitsraum_frei/1(Out1) -> Bus Creator/4  "arbeitsraum_frei"
  zylinder_entfernt_folge/1(Out1) -> Bus Creator/5  "zylinder_entfernt_folge"
  folge_belegt/1(Out1) -> Bus Creator/6  "folge_belegt"
  Mux/1 -> aktoren/1
  Signal Builder10/1(aufzug_abwaerts) -> Data Type Conversion/1  "aufzug_abwaerts"
  Signal Builder10/2(aufzug_aufwaerts) -> Data Type Conversion1/1  "aufzug_aufwaerts"
  Signal Builder10/3(zylinder_ausschieben) -> Data Type Conversion2/1  "zylinder_ausschieben"
  Signal Builder10/4(luft_an) -> Data Type Conversion3/1  "luft_an"
  Signal Builder10/8(station_frei) -> Data Type Conversion7/1  "station_frei"
  Signal Builder10/5(Signal 5) -> Data Type Conversion4/1
  Signal Builder10/6(Signal 6) -> Data Type Conversion5/1
  Signal Builder10/7(Signal 7) -> Data Type Conversion6/1
  aufzug_abwaerts/1(Out1) -> Mux/1
  aufzug_aufwaerts/1(Out1) -> Mux/2
  zylinder_ausschieben/1(Out1) -> Mux/3
  luft_an/1(Out1) -> Mux/4
  out5/1(Out1) -> Mux/5
  out6/1(Out1) -> Mux/6
  out7/1(Out1) -> Mux/7
  station_frei/1(Out1) -> Mux/8
  zylinder_hoehe/1(Out1) -> Bus Creator/3  "zylinder_hoehe"

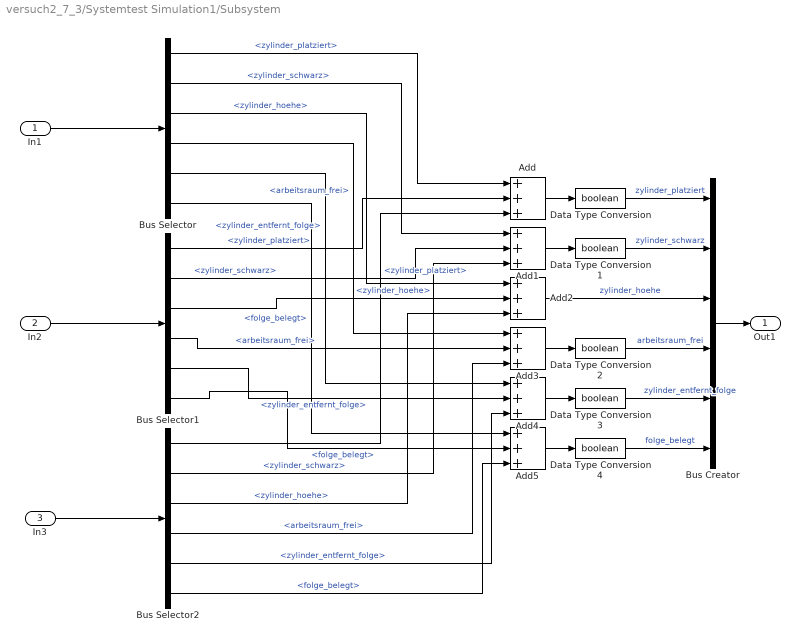
== system versuch2_7_3/Systemtest Simulation1/Subsystem ==
  In1 : Inport
  In2 : Inport  Port=2
  In3 : Inport  Port=3
  Add{,1..5} (6 alike) : Sum  Inputs=+++
  Bus Creator : BusCreator  Inputs=6
  Bus Selector : BusSelector  OutputSignals=zylinder_platziert,zylinder_schwarz,zylinder_hoehe,arbeitsraum_frei,zylinder_entfernt_folge,folge_belegt
  Bus Selector1 : BusSelector  OutputSignals=zylinder_platziert,zylinder_schwarz,zylinder_hoehe,arbeitsraum_frei,zylinder_entfernt_folge,folge_belegt
  Bus Selector2 : BusSelector  OutputSignals=zylinder_platziert,zylinder_schwarz,zylinder_hoehe,arbeitsraum_frei,zylinder_entfernt_folge,folge_belegt
  Data Type Conversion{,1..4} (5 alike) : DataTypeConversion  OutDataTypeStr=boolean
  Out1 : Outport  VectorParamsAs1DForOutWhenUnconnected=off
  wires:
  In1/1 -> Bus Selector/1
  In2/1 -> Bus Selector1/1
  In3/1 -> Bus Selector2/1
  Bus Creator/1 -> Out1/1
  Bus Selector/1 -> Add/1  "<zylinder_platziert>"
  Data Type Conversion/1 -> Bus Creator/1  "zylinder_platziert"
  Bus Selector1/1 -> Add/2  "<zylinder_platziert>"
  Bus Selector2/1 -> Add/3  "<zylinder_platziert>"
  Data Type Conversion1/1 -> Bus Creator/2  "zylinder_schwarz"
  Bus Selector/2 -> Add1/1  "<zylinder_schwarz>"
  Bus Selector1/2 -> Add1/2  "<zylinder_schwarz>"
  Bus Selector2/2 -> Add1/3  "<zylinder_schwarz>"
  Add2/1 -> Bus Creator/3  "zylinder_hoehe"
  Bus Selector/3 -> Add2/1  "<zylinder_hoehe>"
  Bus Selector1/3 -> Add2/2  "<zylinder_hoehe>"
  Bus Selector2/3 -> Add2/3  "<zylinder_hoehe>"
  Add3/1 -> Data Type Conversion2/1
  Bus Selector/4 -> Add3/1  "<arbeitsraum_frei>"
  Bus Selector1/4 -> Add3/2  "<arbeitsraum_frei>"
  Bus Selector2/4 -> Add3/3  "<arbeitsraum_frei>"
  Data Type Conversion3/1 -> Bus Creator/5  "zylinder_entfernt_folge"
  Bus Selector/5 -> Add4/1  "<zylinder_entfernt_folge>"
  Bus Selector1/5 -> Add4/2  "<zylinder_entfernt_folge>"
  Bus Selector2/5 -> Add4/3  "<zylinder_entfernt_folge>"
  Add5/1 -> Data Type Conversion4/1
  Bus Selector/6 -> Add5/1  "<folge_belegt>"
  Bus Selector1/6 -> Add5/2  "<folge_belegt>"
  Bus Selector2/6 -> Add5/3  "<folge_belegt>"
  Add/1 -> Data Type Conversion/1
  Add1/1 -> Data Type Conversion1/1
  Data Type Conversion2/1 -> Bus Creator/4  "arbeitsraum_frei"
  Add4/1 -> Data Type Conversion3/1
  Data Type Conversion4/1 -> Bus Creator/6  "folge_belegt"

== system versuch2_7_3/Systemtest Simulation1/1_schwarz_mit_Deckel/Signal Builder10 ==
  Demux : Demux  Tag=STV Demux  Outputs=8
      settings: DisplayOption=none
  FromWs : FromWorkspace  Tag=STV FromWs  VariableName=tuvar
      SigBuilderData=|
      | common.afterFinalStr = 'Extrapolate'
      | common.sampleTime = 0
      | dataSet.timeRange = [0 11]
      | dataSet.name = 'Group 1'
      | sbobj.Groups.Name = 'Group 1'
      | sbobj.Groups.Signals(1).Name = 'aufzug_abwaerts'
      | sbobj.Groups.Signals(1).XData = [0 6 6 10.5 10.5 11]
      | sbobj.Groups.Signals(1).YData = [0 0 1 1 0 0]
      | sbobj.Groups.Signals(2).Name = 'aufzug_aufwaerts'
      | sbobj.Groups.Signals(2).XData = [0 0.5 0.5 5 5 11]
      | sbobj.Groups.Signals(2).YData = [0 0 1 1 0 0]
      | sbobj.Groups.Signals(3).Name = 'zylinder_ausschieben'
      | sbobj.Groups.Signals(3).XData = [0 5.5 5.5 6.2 6.2 11]
      | sbobj.Groups.Signals(3).YData = [0 0 1 1 0 0]
      | sbobj.Groups.Signals(4).Name = 'luft_an'
      | sbobj.Groups.Signals(4).XData = [0 5.5 5.5 7.5 7.5 11]
      | sbobj.Groups.Signals(4).YData = [0 0 1 1 0 0]
      | sbobj.Groups.Signals(5).Name = 'Signal 5'
      | sbobj.Groups.Signals(5).XData = [0 11]
      | sbobj.Groups.Signals(5).YData = [0 0]
      | sbobj.Groups.Signals(6).Name = 'Signal 6'
      | sbobj.Groups.Signals(6).XData = [0 11]
      | sbobj.Groups.Signals(6).YData = [0 0]
      | sbobj.Groups.Signals(7).Name = 'Signal 7'
      | sbobj.Groups.Signals(7).XData = [0 11]
      | sbobj.Groups.Signals(7).YData = [0 0]
      | sbobj.Groups.Signals(8).Name = 'station_frei'
      | sbobj.Groups.Signals(8).XData = [0 0.1 0.1 11]
      | sbobj.Groups.Signals(8).YData = [1 1 0 0]
      | sbobj.Groups.TimeRange = [0 11]
  aufzug_abwaerts : Outport  Tag=STV Outport  VectorParamsAs1DForOutWhenUnconnected=off
  aufzug_aufwaerts : Outport  Tag=STV Outport  Port=2  VectorParamsAs1DForOutWhenUnconnected=off
  zylinder_ausschieben : Outport  Tag=STV Outport  Port=3  VectorParamsAs1DForOutWhenUnconnected=off
  luft_an : Outport  Tag=STV Outport  Port=4  VectorParamsAs1DForOutWhenUnconnected=off
  Signal 5 : Outport  Tag=STV Outport  Port=5  VectorParamsAs1DForOutWhenUnconnected=off
  Signal 6 : Outport  Tag=STV Outport  Port=6  VectorParamsAs1DForOutWhenUnconnected=off
  Signal 7 : Outport  Tag=STV Outport  Port=7  VectorParamsAs1DForOutWhenUnconnected=off
  station_frei : Outport  Tag=STV Outport  Port=8  VectorParamsAs1DForOutWhenUnconnected=off
  wires:
  Demux/1 -> aufzug_abwaerts/1
  FromWs/1 -> Demux/1
  Demux/2 -> aufzug_aufwaerts/1
  Demux/3 -> zylinder_ausschieben/1
  Demux/4 -> luft_an/1
  Demux/5 -> Signal 5/1
  Demux/6 -> Signal 6/1
  Demux/7 -> Signal 7/1
  Demux/8 -> station_frei/1

== system versuch2_7_3/Systemtest Simulation1/1_schwarz_mit_Deckel/Signal Builder4 ==
  Demux : Demux  Tag=STV Demux  Outputs=6
      settings: DisplayOption=none
  FromWs : FromWorkspace  Tag=STV FromWs  VariableName=tuvar
      SigBuilderData=|
      | common.afterFinalStr = 'Extrapolate'
      | common.sampleTime = 0
      | dataSet.timeRange = [0 11]
      | dataSet.name = 'Group 1'
      | sbobj.Groups.Name = 'Group 1'
      | sbobj.Groups.Signals(1).Name = 'zylinder_platziert'
      | sbobj.Groups.Signals(1).XData = [0 0.3 0.3 11]
      | sbobj.Groups.Signals(1).YData = [1 1 0 0]
      | sbobj.Groups.Signals(2).Name = 'zylinder_schwarz'
      | sbobj.Groups.Signals(2).XData = [0 5.6 5.6 11]
      | sbobj.Groups.Signals(2).YData = [1 1 0 0]
      | sbobj.Groups.Signals(3).Name = 'zylinder_hoehe'
      | sbobj.Groups.Signals(3).XData = [0 5 5 5.6 5.6 11]
      | sbobj.Groups.Signals(3).YData = [0 0 25 25 0 0]
      | sbobj.Groups.Signals(4).Name = 'arbeitsraum_frei'
      | sbobj.Groups.Signals(4).XData = [0 0.5 0.5 10.5 10.5 10.8 10.8 11]
      | sbobj.Groups.Signals(4).YData = [1 1 0 0 1 1 0 0]
      | sbobj.Groups.Signals(5).Name = 'zylinder_entfernt_folge'
      | sbobj.Groups.Signals(5).XData = [0 10 10 10.5 10.5 11]
      | sbobj.Groups.Signals(5).YData = [0 0 1 1 0 0]
      | sbobj.Groups.Signals(6).Name = 'folge_belegt'
      | sbobj.Groups.Signals(6).XData = [0 4 4 5.5 5.5 11]
      | sbobj.Groups.Signals(6).YData = [0 0 1 1 0 0]
      | sbobj.Groups.TimeRange = [0 11]
  zylinder_platziert : Outport  Tag=STV Outport  VectorParamsAs1DForOutWhenUnconnected=off
  zylinder_schwarz : Outport  Tag=STV Outport  Port=2  VectorParamsAs1DForOutWhenUnconnected=off
  zylinder_hoehe : Outport  Tag=STV Outport  Port=3  VectorParamsAs1DForOutWhenUnconnected=off
  arbeitsraum_frei : Outport  Tag=STV Outport  Port=4  VectorParamsAs1DForOutWhenUnconnected=off
  zylinder_entfernt_folge : Outport  Tag=STV Outport  Port=5  VectorParamsAs1DForOutWhenUnconnected=off
  folge_belegt : Outport  Tag=STV Outport  Port=6  VectorParamsAs1DForOutWhenUnconnected=off
  wires:
  Demux/1 -> zylinder_platziert/1
  FromWs/1 -> Demux/1
  Demux/2 -> zylinder_schwarz/1
  Demux/3 -> zylinder_hoehe/1
  Demux/4 -> arbeitsraum_frei/1
  Demux/5 -> zylinder_entfernt_folge/1
  Demux/6 -> folge_belegt/1

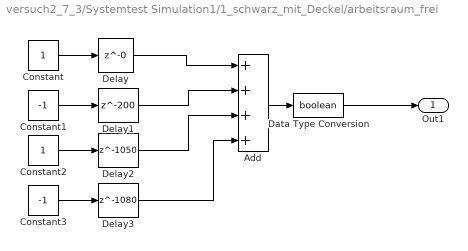
== system versuch2_7_3/Systemtest Simulation1/1_schwarz_mit_Deckel/arbeitsraum_frei ==
  Add : Sum  Inputs=++++
  Constant : Constant
  Constant1 : Constant  Value=-1
  Constant2 : Constant
  Constant3 : Constant  Value=-1
  Data Type Conversion : DataTypeConversion  OutDataTypeStr=boolean
  Delay : Delay  DelayLength=0
  Delay1 : Delay  DelayLength=200
  Delay2 : Delay  DelayLength=1050
  Delay3 : Delay  DelayLength=1080
  Out1 : Outport  VectorParamsAs1DForOutWhenUnconnected=off
  wires:
  Constant/1 -> Delay/1
  Constant1/1 -> Delay1/1
  Delay/1 -> Add/1
  Delay1/1 -> Add/2
  Add/1 -> Data Type Conversion/1
  Data Type Conversion/1 -> Out1/1
  Constant2/1 -> Delay2/1
  Delay2/1 -> Add/3
  Constant3/1 -> Delay3/1
  Delay3/1 -> Add/4

== system versuch2_7_3/Systemtest Simulation1/1_schwarz_mit_Deckel/aufzug_abwaerts ==
  Add : Sum
  Constant : Constant
  Constant1 : Constant  Value=-1
  Data Type Conversion : DataTypeConversion  OutDataTypeStr=boolean
  Delay : Delay  DelayLength=600
  Delay1 : Delay  DelayLength=1050
  Out1 : Outport  VectorParamsAs1DForOutWhenUnconnected=off
  wires:
  Constant/1 -> Delay/1
  Constant1/1 -> Delay1/1
  Delay/1 -> Add/1
  Delay1/1 -> Add/2
  Add/1 -> Data Type Conversion/1
  Data Type Conversion/1 -> Out1/1

== system versuch2_7_3/Systemtest Simulation1/1_schwarz_mit_Deckel/aufzug_aufwaerts ==
  Add : Sum
  Constant : Constant
  Constant1 : Constant  Value=-1
  Data Type Conversion : DataTypeConversion  OutDataTypeStr=boolean
  Delay : Delay  DelayLength=50
  Delay1 : Delay  DelayLength=500
  Out1 : Outport  VectorParamsAs1DForOutWhenUnconnected=off
  wires:
  Constant/1 -> Delay/1
  Constant1/1 -> Delay1/1
  Delay/1 -> Add/1
  Delay1/1 -> Add/2
  Add/1 -> Data Type Conversion/1
  Data Type Conversion/1 -> Out1/1

== system versuch2_7_3/Systemtest Simulation1/1_schwarz_mit_Deckel/done_signal ==
  Constant : Constant
  Data Type Conversion : DataTypeConversion  OutDataTypeStr=boolean
  Delay : Delay  DelayLength=1080
  Out1 : Outport  VectorParamsAs1DForOutWhenUnconnected=off
  wires:
  Constant/1 -> Delay/1
  Data Type Conversion/1 -> Out1/1
  Delay/1 -> Data Type Conversion/1

== system versuch2_7_3/Systemtest Simulation1/1_schwarz_mit_Deckel/folge_belegt ==
  Add : Sum
  Constant1 : Constant
  Constant2 : Constant  Value=-1
  Data Type Conversion1 : DataTypeConversion  OutDataTypeStr=boolean
  Delay : Delay  DelayLength=400
  Delay1 : Delay  DelayLength=550
  Out1 : Outport  VectorParamsAs1DForOutWhenUnconnected=off
  wires:
  Data Type Conversion1/1 -> Out1/1
  Constant1/1 -> Delay/1
  Constant2/1 -> Delay1/1
  Delay/1 -> Add/1
  Delay1/1 -> Add/2
  Add/1 -> Data Type Conversion1/1

== system versuch2_7_3/Systemtest Simulation1/1_schwarz_mit_Deckel/luft_an ==
  Add : Sum
  Constant : Constant
  Constant1 : Constant  Value=-1
  Data Type Conversion : DataTypeConversion  OutDataTypeStr=boolean
  Delay : Delay  DelayLength=550
  Delay1 : Delay  DelayLength=750
  Out1 : Outport  VectorParamsAs1DForOutWhenUnconnected=off
  wires:
  Constant/1 -> Delay/1
  Constant1/1 -> Delay1/1
  Delay/1 -> Add/1
  Delay1/1 -> Add/2
  Add/1 -> Data Type Conversion/1
  Data Type Conversion/1 -> Out1/1

== system versuch2_7_3/Systemtest Simulation1/1_schwarz_mit_Deckel/out5 ==
  Add : Sum
  Constant : Constant
  Constant1 : Constant  Value=-1
  Data Type Conversion : DataTypeConversion  OutDataTypeStr=boolean
  Delay : Delay  DelayLength=0
  Delay1 : Delay  DelayLength=0
  Out1 : Outport  VectorParamsAs1DForOutWhenUnconnected=off
  wires:
  Constant/1 -> Delay/1
  Constant1/1 -> Delay1/1
  Delay/1 -> Add/1
  Delay1/1 -> Add/2
  Add/1 -> Data Type Conversion/1
  Data Type Conversion/1 -> Out1/1

== system versuch2_7_3/Systemtest Simulation1/1_schwarz_mit_Deckel/out6 ==
  Add : Sum
  Constant : Constant
  Constant1 : Constant  Value=-1
  Data Type Conversion : DataTypeConversion  OutDataTypeStr=boolean
  Delay : Delay  DelayLength=0
  Delay1 : Delay  DelayLength=0
  Out1 : Outport  VectorParamsAs1DForOutWhenUnconnected=off
  wires:
  Constant/1 -> Delay/1
  Constant1/1 -> Delay1/1
  Delay/1 -> Add/1
  Delay1/1 -> Add/2
  Add/1 -> Data Type Conversion/1
  Data Type Conversion/1 -> Out1/1

== system versuch2_7_3/Systemtest Simulation1/1_schwarz_mit_Deckel/out7 ==
  Add : Sum
  Constant : Constant
  Constant1 : Constant  Value=-1
  Data Type Conversion : DataTypeConversion  OutDataTypeStr=boolean
  Delay : Delay  DelayLength=0
  Delay1 : Delay  DelayLength=0
  Out1 : Outport  VectorParamsAs1DForOutWhenUnconnected=off
  wires:
  Constant/1 -> Delay/1
  Constant1/1 -> Delay1/1
  Delay/1 -> Add/1
  Delay1/1 -> Add/2
  Add/1 -> Data Type Conversion/1
  Data Type Conversion/1 -> Out1/1

== system versuch2_7_3/Systemtest Simulation1/1_schwarz_mit_Deckel/station_frei ==
  Add : Sum
  Constant : Constant
  Constant1 : Constant  Value=-1
  Data Type Conversion : DataTypeConversion  OutDataTypeStr=boolean
  Delay : Delay  DelayLength=0
  Delay1 : Delay  DelayLength=10
  Out1 : Outport  VectorParamsAs1DForOutWhenUnconnected=off
  wires:
  Constant/1 -> Delay/1
  Constant1/1 -> Delay1/1
  Delay/1 -> Add/1
  Delay1/1 -> Add/2
  Add/1 -> Data Type Conversion/1
  Data Type Conversion/1 -> Out1/1

== system versuch2_7_3/Systemtest Simulation1/1_schwarz_mit_Deckel/zylinder_ausschieben ==
  Add : Sum
  Constant : Constant
  Constant1 : Constant  Value=-1
  Data Type Conversion : DataTypeConversion  OutDataTypeStr=boolean
  Delay : Delay  DelayLength=550
  Delay1 : Delay  DelayLength=620
  Out1 : Outport  VectorParamsAs1DForOutWhenUnconnected=off
  wires:
  Constant/1 -> Delay/1
  Constant1/1 -> Delay1/1
  Delay/1 -> Add/1
  Delay1/1 -> Add/2
  Add/1 -> Data Type Conversion/1
  Data Type Conversion/1 -> Out1/1

== system versuch2_7_3/Systemtest Simulation1/1_schwarz_mit_Deckel/zylinder_entfernt_folge ==
  Add : Sum
  Constant : Constant
  Constant1 : Constant  Value=-1
  Data Type Conversion : DataTypeConversion  OutDataTypeStr=boolean
  Delay : Delay  DelayLength=1000
  Delay1 : Delay  DelayLength=1050
  Out1 : Outport  VectorParamsAs1DForOutWhenUnconnected=off
  wires:
  Constant/1 -> Delay/1
  Constant1/1 -> Delay1/1
  Delay/1 -> Add/1
  Delay1/1 -> Add/2
  Add/1 -> Data Type Conversion/1
  Data Type Conversion/1 -> Out1/1

== system versuch2_7_3/Systemtest Simulation1/1_schwarz_mit_Deckel/zylinder_hoehe ==
  Add : Sum
  Constant : Constant  Value=25
  Constant1 : Constant  Value=-25
  Delay : Delay  DelayLength=50
  Delay1 : Delay  DelayLength=900
  Out1 : Outport  VectorParamsAs1DForOutWhenUnconnected=off
  wires:
  Constant/1 -> Delay/1
  Constant1/1 -> Delay1/1
  Delay/1 -> Add/1
  Delay1/1 -> Add/2
  Add/1 -> Out1/1

== system versuch2_7_3/Systemtest Simulation1/1_schwarz_mit_Deckel/zylinder_platziert ==
  Add : Sum
  Constant : Constant
  Constant1 : Constant  Value=-1
  Data Type Conversion : DataTypeConversion  OutDataTypeStr=boolean
  Delay : Delay  DelayLength=50
  Delay1 : Delay  DelayLength=70
  Out1 : Outport  VectorParamsAs1DForOutWhenUnconnected=off
  wires:
  Constant/1 -> Delay/1
  Constant1/1 -> Delay1/1
  Delay/1 -> Add/1
  Delay1/1 -> Add/2
  Add/1 -> Data Type Conversion/1
  Data Type Conversion/1 -> Out1/1

== system versuch2_7_3/Systemtest Simulation1/1_schwarz_mit_Deckel/zylinder_schwarz ==
  Add : Sum
  Constant : Constant
  Constant1 : Constant  Value=-1
  Data Type Conversion : DataTypeConversion  OutDataTypeStr=boolean
  Delay : Delay  DelayLength=0
  Delay1 : Delay  DelayLength=700
  Out1 : Outport  VectorParamsAs1DForOutWhenUnconnected=off
  wires:
  Constant/1 -> Delay/1
  Constant1/1 -> Delay1/1
  Delay/1 -> Add/1
  Delay1/1 -> Add/2
  Add/1 -> Data Type Conversion/1
  Data Type Conversion/1 -> Out1/1

== system versuch2_7_3/Systemtest Simulation1/2_rot_mit_Deckel/Signal Builder10 ==
  Demux : Demux  Tag=STV Demux  Outputs=8
      settings: DisplayOption=none
  FromWs : FromWorkspace  Tag=STV FromWs  VariableName=tuvar
      SigBuilderData=|
      | common.afterFinalStr = 'Extrapolate'
      | common.sampleTime = 0
      | dataSet.timeRange = [0 11]
      | dataSet.name = 'Group 1'
      | sbobj.Groups.Name = 'Group 1'
      | sbobj.Groups.Signals(1).Name = 'aufzug_abwaerts'
      | sbobj.Groups.Signals(1).XData = [0 6 6 10.5 10.5 11]
      | sbobj.Groups.Signals(1).YData = [0 0 1 1 0 0]
      | sbobj.Groups.Signals(2).Name = 'aufzug_aufwaerts'
      | sbobj.Groups.Signals(2).XData = [0 0.5 0.5 5 5 11]
      | sbobj.Groups.Signals(2).YData = [0 0 1 1 0 0]
      | sbobj.Groups.Signals(3).Name = 'zylinder_ausschieben'
      | sbobj.Groups.Signals(3).XData = [0 5.5 5.5 6.2 6.2 11]
      | sbobj.Groups.Signals(3).YData = [0 0 1 1 0 0]
      | sbobj.Groups.Signals(4).Name = 'luft_an'
      | sbobj.Groups.Signals(4).XData = [0 5.5 5.5 7.5 7.5 11]
      | sbobj.Groups.Signals(4).YData = [0 0 1 1 0 0]
      | sbobj.Groups.Signals(5).Name = 'Signal 5'
      | sbobj.Groups.Signals(5).XData = [0 11]
      | sbobj.Groups.Signals(5).YData = [0 0]
      | sbobj.Groups.Signals(6).Name = 'Signal 6'
      | sbobj.Groups.Signals(6).XData = [0 11]
      | sbobj.Groups.Signals(6).YData = [0 0]
      | sbobj.Groups.Signals(7).Name = 'Signal 7'
      | sbobj.Groups.Signals(7).XData = [0 11]
      | sbobj.Groups.Signals(7).YData = [0 0]
      | sbobj.Groups.Signals(8).Name = 'station_frei'
      | sbobj.Groups.Signals(8).XData = [0 0.1 0.1 11]
      | sbobj.Groups.Signals(8).YData = [1 1 0 0]
      | sbobj.Groups.TimeRange = [0 11]
  aufzug_abwaerts : Outport  Tag=STV Outport  VectorParamsAs1DForOutWhenUnconnected=off
  aufzug_aufwaerts : Outport  Tag=STV Outport  Port=2  VectorParamsAs1DForOutWhenUnconnected=off
  zylinder_ausschieben : Outport  Tag=STV Outport  Port=3  VectorParamsAs1DForOutWhenUnconnected=off
  luft_an : Outport  Tag=STV Outport  Port=4  VectorParamsAs1DForOutWhenUnconnected=off
  Signal 5 : Outport  Tag=STV Outport  Port=5  VectorParamsAs1DForOutWhenUnconnected=off
  Signal 6 : Outport  Tag=STV Outport  Port=6  VectorParamsAs1DForOutWhenUnconnected=off
  Signal 7 : Outport  Tag=STV Outport  Port=7  VectorParamsAs1DForOutWhenUnconnected=off
  station_frei : Outport  Tag=STV Outport  Port=8  VectorParamsAs1DForOutWhenUnconnected=off
  wires:
  Demux/1 -> aufzug_abwaerts/1
  FromWs/1 -> Demux/1
  Demux/2 -> aufzug_aufwaerts/1
  Demux/3 -> zylinder_ausschieben/1
  Demux/4 -> luft_an/1
  Demux/5 -> Signal 5/1
  Demux/6 -> Signal 6/1
  Demux/7 -> Signal 7/1
  Demux/8 -> station_frei/1

== system versuch2_7_3/Systemtest Simulation1/2_rot_mit_Deckel/Signal Builder4 ==
  Demux : Demux  Tag=STV Demux  Outputs=6
      settings: DisplayOption=none
  FromWs : FromWorkspace  Tag=STV FromWs  VariableName=tuvar
      SigBuilderData=|
      | common.afterFinalStr = 'Extrapolate'
      | common.sampleTime = 0
      | dataSet.timeRange = [0 11]
      | dataSet.name = 'Group 1'
      | sbobj.Groups.Name = 'Group 1'
      | sbobj.Groups.Signals(1).Name = 'zylinder_platziert'
      | sbobj.Groups.Signals(1).XData = [0 0.3 0.3 11]
      | sbobj.Groups.Signals(1).YData = [1 1 0 0]
      | sbobj.Groups.Signals(2).Name = 'zylinder_schwarz'
      | sbobj.Groups.Signals(2).XData = [0 11]
      | sbobj.Groups.Signals(2).YData = [0 0]
      | sbobj.Groups.Signals(3).Name = 'zylinder_hoehe'
      | sbobj.Groups.Signals(3).XData = [0 5 5 5.6 5.6 11]
      | sbobj.Groups.Signals(3).YData = [0 0 28 28 0 0]
      | sbobj.Groups.Signals(4).Name = 'arbeitsraum_frei'
      | sbobj.Groups.Signals(4).XData = [0 0.5 0.5 10.5 10.5 10.8 10.8 11]
      | sbobj.Groups.Signals(4).YData = [1 1 0 0 1 1 0 0]
      | sbobj.Groups.Signals(5).Name = 'zylinder_entfernt_folge'
      | sbobj.Groups.Signals(5).XData = [0 10 10 10.5 10.5 11]
      | sbobj.Groups.Signals(5).YData = [0 0 1 1 0 0]
      | sbobj.Groups.Signals(6).Name = 'folge_belegt'
      | sbobj.Groups.Signals(6).XData = [0 4 5.5 11]
      | sbobj.Groups.Signals(6).YData = [0 0 0 0]
      | sbobj.Groups.TimeRange = [0 11]
  zylinder_platziert : Outport  Tag=STV Outport  VectorParamsAs1DForOutWhenUnconnected=off
  zylinder_schwarz : Outport  Tag=STV Outport  Port=2  VectorParamsAs1DForOutWhenUnconnected=off
  zylinder_hoehe : Outport  Tag=STV Outport  Port=3  VectorParamsAs1DForOutWhenUnconnected=off
  arbeitsraum_frei : Outport  Tag=STV Outport  Port=4  VectorParamsAs1DForOutWhenUnconnected=off
  zylinder_entfernt_folge : Outport  Tag=STV Outport  Port=5  VectorParamsAs1DForOutWhenUnconnected=off
  folge_belegt : Outport  Tag=STV Outport  Port=6  VectorParamsAs1DForOutWhenUnconnected=off
  wires:
  Demux/1 -> zylinder_platziert/1
  FromWs/1 -> Demux/1
  Demux/2 -> zylinder_schwarz/1
  Demux/3 -> zylinder_hoehe/1
  Demux/4 -> arbeitsraum_frei/1
  Demux/5 -> zylinder_entfernt_folge/1
  Demux/6 -> folge_belegt/1

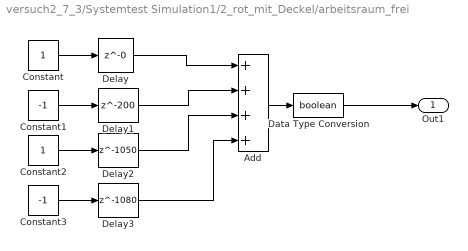
== system versuch2_7_3/Systemtest Simulation1/2_rot_mit_Deckel/arbeitsraum_frei ==
  Add : Sum  Inputs=++++
  Constant : Constant
  Constant1 : Constant  Value=-1
  Constant2 : Constant
  Constant3 : Constant  Value=-1
  Data Type Conversion : DataTypeConversion  OutDataTypeStr=boolean
  Delay : Delay  DelayLength=0
  Delay1 : Delay  DelayLength=200
  Delay2 : Delay  DelayLength=1050
  Delay3 : Delay  DelayLength=1080
  Out1 : Outport  VectorParamsAs1DForOutWhenUnconnected=off
  wires:
  Constant/1 -> Delay/1
  Constant1/1 -> Delay1/1
  Delay/1 -> Add/1
  Delay1/1 -> Add/2
  Add/1 -> Data Type Conversion/1
  Data Type Conversion/1 -> Out1/1
  Constant2/1 -> Delay2/1
  Delay2/1 -> Add/3
  Constant3/1 -> Delay3/1
  Delay3/1 -> Add/4

== system versuch2_7_3/Systemtest Simulation1/2_rot_mit_Deckel/aufzug_abwaerts ==
  Add : Sum
  Constant : Constant
  Constant1 : Constant  Value=-1
  Data Type Conversion : DataTypeConversion  OutDataTypeStr=boolean
  Delay : Delay  DelayLength=600
  Delay1 : Delay  DelayLength=1050
  Out1 : Outport  VectorParamsAs1DForOutWhenUnconnected=off
  wires:
  Constant/1 -> Delay/1
  Constant1/1 -> Delay1/1
  Delay/1 -> Add/1
  Delay1/1 -> Add/2
  Add/1 -> Data Type Conversion/1
  Data Type Conversion/1 -> Out1/1

== system versuch2_7_3/Systemtest Simulation1/2_rot_mit_Deckel/aufzug_aufwaerts ==
  Add : Sum
  Constant : Constant
  Constant1 : Constant  Value=-1
  Data Type Conversion : DataTypeConversion  OutDataTypeStr=boolean
  Delay : Delay  DelayLength=50
  Delay1 : Delay  DelayLength=500
  Out1 : Outport  VectorParamsAs1DForOutWhenUnconnected=off
  wires:
  Constant/1 -> Delay/1
  Constant1/1 -> Delay1/1
  Delay/1 -> Add/1
  Delay1/1 -> Add/2
  Add/1 -> Data Type Conversion/1
  Data Type Conversion/1 -> Out1/1

== system versuch2_7_3/Systemtest Simulation1/2_rot_mit_Deckel/done_signal ==
  Constant : Constant
  Data Type Conversion : DataTypeConversion  OutDataTypeStr=boolean
  Delay : Delay  DelayLength=1080
  Out1 : Outport  VectorParamsAs1DForOutWhenUnconnected=off
  wires:
  Constant/1 -> Delay/1
  Data Type Conversion/1 -> Out1/1
  Delay/1 -> Data Type Conversion/1

== system versuch2_7_3/Systemtest Simulation1/2_rot_mit_Deckel/folge_belegt ==
  Constant : Constant  Value=0
  Data Type Conversion : DataTypeConversion  OutDataTypeStr=boolean
  Out1 : Outport  VectorParamsAs1DForOutWhenUnconnected=off
  wires:
  Constant/1 -> Data Type Conversion/1
  Data Type Conversion/1 -> Out1/1
